simulink model "SAS"  (R2016a)
settings: Solver=ode45  SolverMode=SingleTasking  StartTime=0.0  StopTime=10.0  RelTol=1e-3  AbsTol=1e-6
values from neighbouring files (symbols this model uses):
  ADC_V2C = 2^16/40    (= 1638.4)    [run_SAS_NB.m]
  Coil = containers.Map    [run_SAS_NB.m]
  DAC_C2V = 20/2^16    (= 0.00030517578125)    [run_SAS_NB.m]
  Elec = containers.Map    [run_SAS_NB.m]
  Filt = containers.Map    [run_SAS_NB.m]
  gradvari = 0.1    [run_SAS_NB.m]
  IMCoilN = 2    [run_SAS_NB.m]
  Magnet = containers.Map    [run_SAS_NB.m]
  magvari = 0.2    [run_SAS_NB.m]
  MNCoilN = 2    [run_SAS_NB.m]
  Noise = containers.Map    [run_SAS_NB.m]
  Susp = containers.Map    [run_SAS_NB.m]
  SW = ones(1,length(loopNames))    [run_SAS_NB.m]
  TMCoilN = 4    [run_SAS_NB.m]
  VertCoup = 0.01    [run_SAS_NB.m]
libraries: cstblocks x26, NbLibrary x22
CloseFcn:
  | ;slview('closediagram',bdroot);
settings Model: SimulationMode=external  ExtModeTrigMode=oneshot  ExtModeArmWhenConnect=off  Creator=controls  LastModifiedBy=yuta
settings DataIOCC: SaveFormat=Array  SignalLoggingSaveFormat=ModelDataLogs
settings OptimizationCC: BlockReduction=off  BooleanDataType=off
settings DebuggingCC: SaveWithParameterizedLinksMsg=none  UnderspecifiedInitializationDetection=Classic  MergeDetectMultiDrivingBlocksExec=none  SignalResolutionControl=TryResolveAllWithWarning  MultiTaskDSMMsg=warning  MultiTaskCondExecSysMsg=none  StateNameClashWarn=warning
settings HardwareCC: ProdBitPerPointer=32  ProdLargestAtomicFloat=None  ProdIntDivRoundTo=Undefined  ProdEndianess=Unspecified  ProdWordSize=32  ProdHWDeviceType=32-bit Generic  TargetUnknown=on
settings ModelReferenceCC: PropagateSignalLabelsOutOfModel=off
settings RTWCC: TemplateMakefile=grt_unix.tmf
settings GRTTargetCC: CombineOutputUpdateFcns=off  GRTInterface=on
settings ConfigComp: CovModelRefEnable=Off  CovSFcnEnable=off

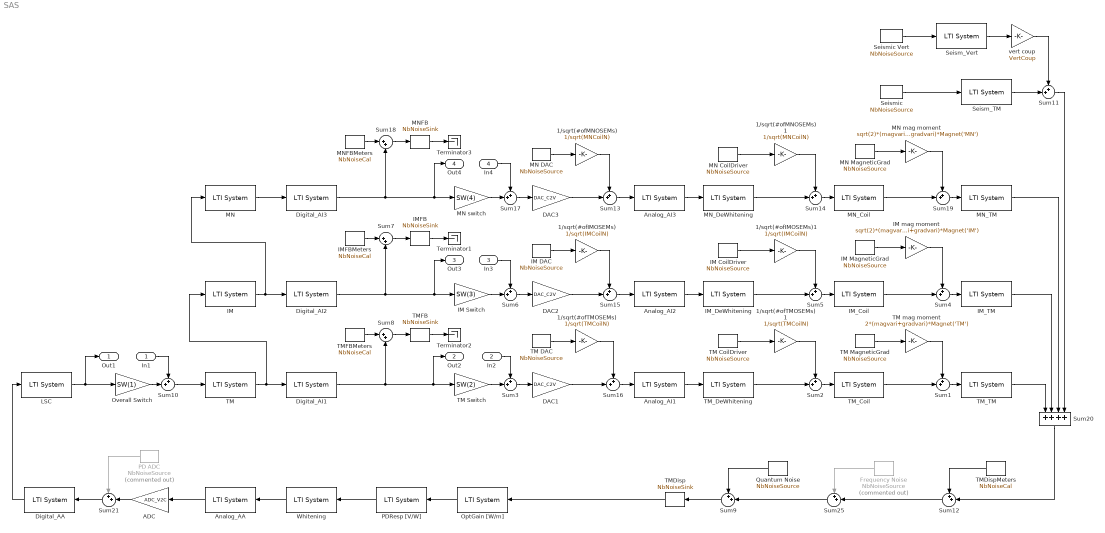
== system SAS ==
  In1 : Inport
  In2 : Inport  Port=2
  In3 : Inport  Port=3
  In4 : Inport  Port=4
  1/sqrt(#ofIMOSEMs) : Gain  Gain=1/sqrt(IMCoilN)
  1/sqrt(#ofIMOSEMs)1 : Gain  Gain=1/sqrt(IMCoilN)
  1/sqrt(#ofMNOSEMs) : Gain  Gain=1/sqrt(MNCoilN)
  1/sqrt(#ofMNOSEMs)1 : Gain  Gain=1/sqrt(MNCoilN)
  1/sqrt(#ofTMOSEMs) : Gain  Gain=1/sqrt(TMCoilN)
  1/sqrt(#ofTMOSEMs)1 : Gain  Gain=1/sqrt(TMCoilN)
  ADC : Gain  Gain=ADC_V2C  SaturateOnIntegerOverflow=on  OutDataTypeStr=Inherit: Same as input  ParamDataTypeStr=Inherit: Same as input
  Analog_AA : cstblocks/LTI System  sys=Elec('Analog_AI')  IC=[]
  Analog_AI1 : cstblocks/LTI System  sys=Elec('Analog_AI')  IC=[]
  Analog_AI2 : cstblocks/LTI System  sys=Elec('Analog_AI')  IC=[]
  Analog_AI3 : cstblocks/LTI System  sys=Elec('Analog_AI')  IC=[]
  DAC1 : Gain  Gain=DAC_C2V  SaturateOnIntegerOverflow=on  OutDataTypeStr=Inherit: Same as input  ParamDataTypeStr=Inherit: Same as input
  DAC2 : Gain  Gain=DAC_C2V  SaturateOnIntegerOverflow=on  OutDataTypeStr=Inherit: Same as input  ParamDataTypeStr=Inherit: Same as input
  DAC3 : Gain  Gain=DAC_C2V  SaturateOnIntegerOverflow=on  OutDataTypeStr=Inherit: Same as input  ParamDataTypeStr=Inherit: Same as input
  Digital_AA : cstblocks/LTI System  sys=Elec('Digital_AI')  IC=[]
  Digital_AI1 : cstblocks/LTI System  sys=Elec('Digital_AI')  IC=[]
  Digital_AI2 : cstblocks/LTI System  sys=Elec('Digital_AI')  IC=[]
  Digital_AI3 : cstblocks/LTI System  sys=Elec('Digital_AI')  IC=[]
  Frequency Noise : NbLibrary/NbNoiseSource  Tag=NbNoiseSource  Commented=on  asd=Noise('Frequency')  chan=''  groupNest=1  group='Frequency noise'  subgroup=''  subsubgroup=''  subsubsubgroup=''
      settings: AttributesFormatString=%<Tag>
  IM : cstblocks/LTI System  sys=Filt('IM')  IC=[]
  IM CoilDriver : NbLibrary/NbNoiseSource  Tag=NbNoiseSource  asd=Noise('IM_Coil')  chan=''  groupNest=1  group='Actuator noise'  subgroup=''  subsubgroup=''  subsubsubgroup=''
      settings: AttributesFormatString=%<Tag>
  IM DAC : NbLibrary/NbNoiseSource  Tag=NbNoiseSource  asd=Noise('DAC')  chan=''  groupNest=1  group='Actuator noise'  subgroup=''  subsubgroup=''  subsubsubgroup=''
      settings: AttributesFormatString=%<Tag>
  IM MagneticGrad : NbLibrary/NbNoiseSource  Tag=NbNoiseSource  asd=Noise('MagneticGradient')  chan=''  groupNest=1  group='Magnetic noise'  subgroup=''  subsubgroup=''  subsubsubgroup=''
      settings: AttributesFormatString=%<Tag>
  IM Switch : Gain  Gain=SW(3)
  IM mag moment : Gain  Gain=sqrt(2)*(magvari+gradvari)*Magnet('IM')
  IMFB : NbLibrary/NbNoiseSink  Tag=NbNoiseSink  dof='IMFB'  asd=DAC_Range  chan=''
      settings: AttributesFormatString=%<Tag>
  IMFBMeters : NbLibrary/NbNoiseCal  Tag=NbNoiseCal  dof='IMFB'  unit='DAC output [cnt/rtHz]'
      settings: AttributesFormatString=%<Tag>
  IM_Coil : cstblocks/LTI System  sys=Coil('IM')  IC=[]
  IM_DeWhitening : cstblocks/LTI System  sys=Elec('IM_DeWhitening')  IC=[]
  IM_TM : cstblocks/LTI System  Description=FlexTf: Susp('IM_TM')  sys=Susp('IM_TM_fit')  IC=[]
      settings: AttributesFormatString=%<Description>
  LSC : cstblocks/LTI System  sys=Filt('LSC')  IC=[]
  MN : cstblocks/LTI System  sys=Filt('MN')  IC=[]
  MN CoilDriver : NbLibrary/NbNoiseSource  Tag=NbNoiseSource  asd=Noise('MN_Coil')  chan=''  groupNest=1  group='Actuator noise'  subgroup=''  subsubgroup=''  subsubsubgroup=''
      settings: AttributesFormatString=%<Tag>
  MN DAC : NbLibrary/NbNoiseSource  Tag=NbNoiseSource  asd=Noise('DAC')  chan=''  groupNest=1  group='Actuator noise'  subgroup=''  subsubgroup=''  subsubsubgroup=''
      settings: AttributesFormatString=%<Tag>
  MN MagneticGrad : NbLibrary/NbNoiseSource  Tag=NbNoiseSource  asd=Noise('MagneticGradient')  chan=''  groupNest=1  group='Magnetic noise'  subgroup=''  subsubgroup=''  subsubsubgroup=''
      settings: AttributesFormatString=%<Tag>
  MN mag moment : Gain  Gain=sqrt(2)*(magvari+gradvari)*Magnet('MN')
  MN switch : Gain  Gain=SW(4)
  MNFB : NbLibrary/NbNoiseSink  Tag=NbNoiseSink  dof='MNFB'  asd=DAC_Range  chan=''
      settings: AttributesFormatString=%<Tag>
  MNFBMeters : NbLibrary/NbNoiseCal  Tag=NbNoiseCal  dof='MNFB'  unit='DAC output [cnt/rtHz]'
      settings: AttributesFormatString=%<Tag>
  MN_Coil : cstblocks/LTI System  sys=Coil('MN')  IC=[]
  MN_DeWhitening : cstblocks/LTI System  sys=Elec('MN_DeWhitening')  IC=[]
  MN_TM : cstblocks/LTI System  Description=FlexTf: Susp('MN_TM')  sys=Susp('MN_TM_fit')  IC=[]
      settings: AttributesFormatString=%<Description>
  OptGain [W/m] : cstblocks/LTI System  sys=OptGain  IC=[]
  Overall Switch : Gain  Gain=SW(1)
  PD ADC : NbLibrary/NbNoiseSource  Tag=NbNoiseSource  Commented=on  asd=Noise('ADC')  chan=''  groupNest=1  group='Sensor noise'  subgroup=''  subsubgroup=''  subsubsubgroup=''
      settings: AttributesFormatString=%<Tag>
  PDResp [V/W] : cstblocks/LTI System  sys=PDResp  IC=[]
  Quantum Noise : NbLibrary/NbNoiseSource  Tag=NbNoiseSource  asd=Noise('Quantum')  chan=''  groupNest=1  group='Quantum noise'  subgroup=''  subsubgroup=''  subsubsubgroup=''
      settings: AttributesFormatString=%<Tag>
  Seism_TM : cstblocks/LTI System  Description=FlexTf: Susp('Seism_TM')  sys=1  IC=[]
      settings: AttributesFormatString=%<Description>
  Seism_Vert : cstblocks/LTI System  Description=FlexTf: Susp('Seism_Vert')  sys=1  IC=[]
      settings: AttributesFormatString=%<Description>
  Seismic : NbLibrary/NbNoiseSource  Tag=NbNoiseSource  asd=Noise('Seismic')  chan=''  groupNest=1  group='Seismic noise'  subgroup=''  subsubgroup=''  subsubsubgroup=''
      settings: AttributesFormatString=%<Tag>
  Seismic Vert : NbLibrary/NbNoiseSource  Tag=NbNoiseSource  asd=Noise('Seismic')  chan=''  groupNest=1  group='Seismic noise'  subgroup=''  subsubgroup=''  subsubsubgroup=''
      settings: AttributesFormatString=%<Tag>
  Sum{1..6,9..17,19,21,25} (18 alike) : Sum  Inputs=++|
  Sum18 : Sum  Inputs=|++
  Sum20 : Sum  Inputs=++++
  Sum7 : Sum  Inputs=|++
  Sum8 : Sum  Inputs=|++
  TM : cstblocks/LTI System  sys=Filt('TM')  IC=[]
  TM CoilDriver : NbLibrary/NbNoiseSource  Tag=NbNoiseSource  asd=Noise('TM_Coil')  chan=''  groupNest=1  group='Actuator noise'  subgroup=''  subsubgroup=''  subsubsubgroup=''
      settings: AttributesFormatString=%<Tag>
  TM DAC : NbLibrary/NbNoiseSource  Tag=NbNoiseSource  asd=Noise('DAC')  chan=''  groupNest=1  group='Actuator noise'  subgroup=''  subsubgroup=''  subsubsubgroup=''
      settings: AttributesFormatString=%<Tag>
  TM MagneticGrad : NbLibrary/NbNoiseSource  Tag=NbNoiseSource  asd=Noise('MagneticGradient')  chan=''  groupNest=1  group='Magnetic noise'  subgroup=''  subsubgroup=''  subsubsubgroup=''
      settings: AttributesFormatString=%<Tag>
  TM Switch : Gain  Gain=SW(2)
  TM mag moment : Gain  Gain=2*(magvari+gradvari)*Magnet('TM')
  TMDisp : NbLibrary/NbNoiseSink  Tag=NbNoiseSink  dof='TMDisp'  asd=0  chan=''
      settings: AttributesFormatString=%<Tag>
  TMDispMeters : NbLibrary/NbNoiseCal  Tag=NbNoiseCal  dof='TMDisp'  unit='TM displacement [m/rtHz]'
      settings: AttributesFormatString=%<Tag>
  TMFB : NbLibrary/NbNoiseSink  Tag=NbNoiseSink  dof='TMFB'  asd=DAC_Range  chan=''
      settings: AttributesFormatString=%<Tag>
  TMFBMeters : NbLibrary/NbNoiseCal  Tag=NbNoiseCal  dof='TMFB'  unit='DAC output [cnt/rtHz]'
      settings: AttributesFormatString=%<Tag>
  TM_Coil : cstblocks/LTI System  sys=Coil('TM')  IC=[]
  TM_DeWhitening : cstblocks/LTI System  sys=Elec('TM_DeWhitening')  IC=[]
  TM_TM : cstblocks/LTI System  Description=FlexTf: Susp('TM_TM')  sys=Susp('TM_TM_fit')  IC=[]
      settings: AttributesFormatString=%<Description>
  Terminator1 : Terminator
  Terminator2 : Terminator
  Terminator3 : Terminator
  Whitening : cstblocks/LTI System  sys=Elec('Whitening')  IC=[]
  vert coup : Gain  Gain=VertCoup
  Out1 : Outport
  Out2 : Outport  Port=2
  Out3 : Outport  Port=3
  Out4 : Outport  Port=4
  wires:
  TM CoilDriver/1 -> 1/sqrt(#ofTMOSEMs)1/1
  Sum2/1 -> TM_Coil/1
  IM CoilDriver/1 -> 1/sqrt(#ofIMOSEMs)1/1
  IM_DeWhitening/1 -> Sum5/2
  Sum5/1 -> IM_Coil/1
  Analog_AI2/1 -> IM_DeWhitening/1
  DAC2/1 -> Sum15/2
  Sum15/1 -> Analog_AI2/1
  DAC1/1 -> Sum16/2
  Sum16/1 -> Analog_AI1/1
  IM/1 -> Digital_AI2/1, MN/1
  TM/1 -> Digital_AI1/1, IM/1
  IMFBMeters/1 -> Sum7/1
  Digital_AI2/1 -> Sum7/2, Out3/1, IM Switch/1
  Sum6/1 -> DAC2/1
  TMFBMeters/1 -> Sum8/1
  Sum3/1 -> DAC1/1
  Digital_AI1/1 -> Sum8/2, Out2/1, TM Switch/1
  TM Switch/1 -> Sum3/2
  In2/1 -> Sum3/1
  IM Switch/1 -> Sum6/2
  In3/1 -> Sum6/1
  Seismic/1 -> Seism_TM/1
  Seism_TM/1 -> Sum11/2
  TM DAC/1 -> 1/sqrt(#ofTMOSEMs)/1
  1/sqrt(#ofTMOSEMs)/1 -> Sum16/1
  IM DAC/1 -> 1/sqrt(#ofIMOSEMs)/1
  1/sqrt(#ofIMOSEMs)/1 -> Sum15/1
  1/sqrt(#ofIMOSEMs)1/1 -> Sum5/1
  1/sqrt(#ofTMOSEMs)1/1 -> Sum2/1
  Seism_Vert/1 -> vert coup/1
  Seismic Vert/1 -> Seism_Vert/1
  vert coup/1 -> Sum11/1
  Sum7/1 -> IMFB/1
  IMFB/1 -> Terminator1/1
  Sum8/1 -> TMFB/1
  TMFB/1 -> Terminator2/1
  Quantum Noise/1 -> Sum9/1
  MN CoilDriver/1 -> 1/sqrt(#ofMNOSEMs)1/1
  MN_DeWhitening/1 -> Sum14/2
  Sum14/1 -> MN_Coil/1
  Analog_AI3/1 -> MN_DeWhitening/1
  DAC3/1 -> Sum13/2
  Sum13/1 -> Analog_AI3/1
  MN/1 -> Digital_AI3/1
  MNFBMeters/1 -> Sum18/1
  Digital_AI3/1 -> Sum18/2, Out4/1, MN switch/1
  Sum17/1 -> DAC3/1
  MN switch/1 -> Sum17/2
  In4/1 -> Sum17/1
  MN DAC/1 -> 1/sqrt(#ofMNOSEMs)/1
  1/sqrt(#ofMNOSEMs)/1 -> Sum13/1
  1/sqrt(#ofMNOSEMs)1/1 -> Sum14/1
  Sum18/1 -> MNFB/1
  MNFB/1 -> Terminator3/1
  TM_TM/1 -> Sum20/1
  IM_TM/1 -> Sum20/2
  MN_TM/1 -> Sum20/3
  Sum1/1 -> TM_TM/1
  TM_Coil/1 -> Sum1/2
  TM MagneticGrad/1 -> TM mag moment/1
  TM mag moment/1 -> Sum1/1
  Sum4/1 -> IM_TM/1
  IM_Coil/1 -> Sum4/2
  IM MagneticGrad/1 -> IM mag moment/1
  IM mag moment/1 -> Sum4/1
  Sum19/1 -> MN_TM/1
  MN_Coil/1 -> Sum19/2
  MN MagneticGrad/1 -> MN mag moment/1
  MN mag moment/1 -> Sum19/1
  Sum11/1 -> Sum20/4
  TMDispMeters/1 -> Sum12/1
  Sum9/1 -> TMDisp/1
  Frequency Noise/1 -> Sum25/1
  Sum25/1 -> Sum9/2
  Sum20/1 -> Sum12/2
  Sum12/1 -> Sum25/2
  TMDisp/1 -> OptGain [W/m]/1
  Analog_AI1/1 -> TM_DeWhitening/1
  TM_DeWhitening/1 -> Sum2/2
  Whitening/1 -> Analog_AA/1
  Analog_AA/1 -> ADC/1
  Overall Switch/1 -> Sum10/2
  In1/1 -> Sum10/1
  Sum10/1 -> TM/1
  LSC/1 -> Out1/1, Overall Switch/1
  Digital_AA/1 -> LSC/1
  PDResp [V/W]/1 -> Whitening/1
  OptGain [W/m]/1 -> PDResp [V/W]/1
  ADC/1 -> Sum21/2
  Sum21/1 -> Digital_AA/1
  PD ADC/1 -> Sum21/1
